simulink model "HPF_V01"  (R2018b)
settings: Solver=ode45  StartTime=0.0  StopTime=0.1  MaxStep=1e-6  RelTol=1e-3  EnableMultiTasking=on
libraries: fl_lib x18, nesl_utility x4, simulink x1
Description:
  | Inverting Op-Amp Circuit
  | 
  | This model shows a standard inverting op-amp circuit. The gain is given by -R2/R1, and
  | with the values set to R1=1K Ohm and R2=10K Ohm, the 0.1V peak-to-peak input
  | voltage is amplified to 1V peak-to-peak. As the Op-Amp block implements an ideal
  | (i.e. infinite gain) device, this gain is achieved regardless of output load.
  | 
  | 
  | Copyright 2008-2015 The MathWorks, Inc.
settings Model: ExtModeAutoUpdateStatusClock=off  Creator=MathWorks  LastModifiedBy=arkad
settings DataIOCC: LimitDataPoints=on  SaveFormat=Array  SignalLoggingSaveFormat=ModelDataLogs
settings OptimizationCC: ExpressionDepthLimit=2147483647  InitFltsAndDblsToZero=on  EfficientMapNaN2IntZero=off  LifeSpan=inf
settings DebuggingCC: SaveWithParameterizedLinksMsg=none  UnderspecifiedInitializationDetection=Classic  MergeDetectMultiDrivingBlocksExec=none  SignalResolutionControl=TryResolveAllWithWarning  SolverPrmCheckMsg=warning  FcnCallInpInsideContextMsg=warning  StateNameClashWarn=warning  SFUnexpectedBacktrackingDiag=warning  SFNoUnconditionalDefaultTransitionDiag=warning  SFExecutionAtInitializationDiag=none
settings HardwareCC: ProdBitPerPointer=32  ProdBitPerSizeT=32  ProdBitPerPtrDiffT=32  ProdLargestAtomicFloat=None  ProdIntDivRoundTo=Undefined  ProdEndianess=Unspecified  ProdWordSize=32  ProdHWDeviceType=32-bit Generic
settings ModelReferenceCC: PropagateSignalLabelsOutOfModel=off
settings SFSimCC: SimUseLocalCustomCode=off
settings RTWCC: RTWUseLocalCustomCode=off
settings CodeAppCC: StateflowObjectComments=on
settings GRTTargetCC: TargetFcnLib=ansi_tfl_tmw.mat  TargetLangStandard=C89/C90 (ANSI)  GeneratePreprocessorConditionals=Disable all  CombineOutputUpdateFcns=off  GRTInterface=on
settings ConfigComp: CovMetricSettings=dw  CovHtmlReporting=on  CovSaveCumulativeToWorkspaceVar=on  CovSaveSingleToWorkspaceVar=on  CovExternalEMLEnable=off
settings SimscapeCC: ExplicitSolverDiagnosticOptions=none  SimscapeNormalizeSystem=off

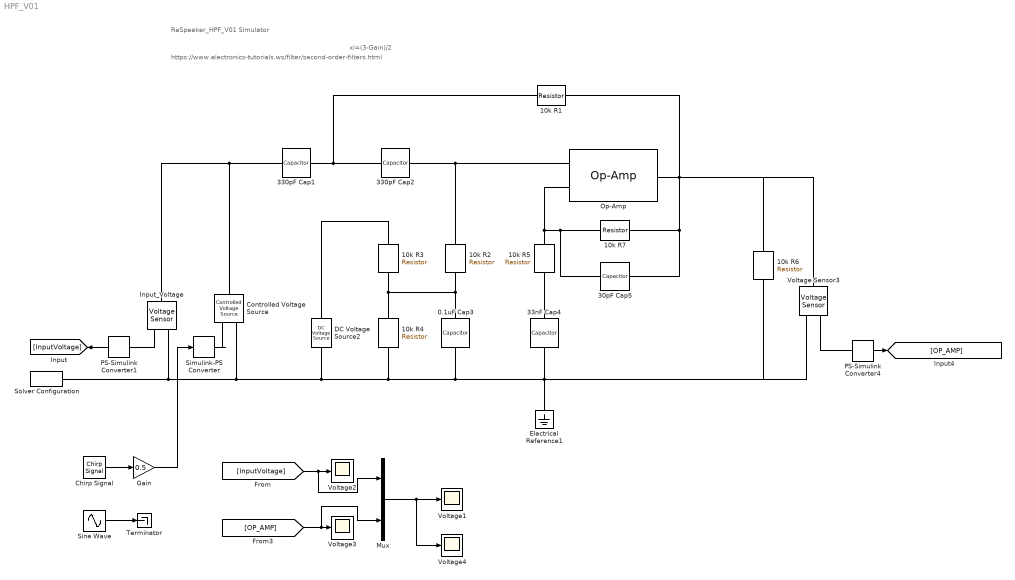
== system HPF_V01 ==
  note: https://www.electronics-tutorials.ws/filter/second-order-filters.html
  note: xi=(3-Gain)/2
  note: ReSpeaker_HPF_V01 Simulator
  0.1uF Cap3 : fl_lib/Electrical/Electrical Elements/Capacitor  c=0.1 uF  r=1e-6 Ohm  g=0 1/Ohm  i_specify=off  i_priority=None  i=0 A  i_nominal_specify=off  i_nominal_unit=A  i_nominal_value=1  v_specify=on  v_priority=None  v=2 V  v_nominal_specify=off  v_nominal_unit=V  v_nominal_value=1  vc_specify=off  vc_priority=High  vc=0 V  vc_nominal_specify=off  vc_nominal_unit=V  vc_nominal_value=1
  10k R{1..6} (6 alike) : fl_lib/Electrical/Electrical Elements/Resistor  R=10 kOhm  i_specify=off  i_priority=High  i=0 A  i_nominal_specify=off  i_nominal_unit=A  i_nominal_value=1  v_specify=off  v_priority=High  v=0 V  v_nominal_specify=off  v_nominal_unit=V  v_nominal_value=1
  10k R7 : fl_lib/Electrical/Electrical Elements/Resistor  R=18 kOhm  i_specify=off  i_priority=High  i=0 A  i_nominal_specify=off  i_nominal_unit=A  i_nominal_value=1  v_specify=off  v_priority=High  v=0 V  v_nominal_specify=off  v_nominal_unit=V  v_nominal_value=1
  30pF Cap5 : fl_lib/Electrical/Electrical Elements/Capacitor  c=30 pF  r=1e-6 Ohm  g=0 1/Ohm  i_specify=off  i_priority=None  i=0 A  i_nominal_specify=off  i_nominal_unit=A  i_nominal_value=1  v_specify=off  v_priority=None  v=0 V  v_nominal_specify=off  v_nominal_unit=V  v_nominal_value=1  vc_specify=off  vc_priority=High  vc=0 V  vc_nominal_specify=off  vc_nominal_unit=V  vc_nominal_value=1
  330pF Cap1 : fl_lib/Electrical/Electrical Elements/Capacitor  c=330 pF  r=1e-6 Ohm  g=0 1/Ohm  i_specify=off  i_priority=None  i=0 A  i_nominal_specify=off  i_nominal_unit=A  i_nominal_value=1  v_specify=off  v_priority=None  v=0 V  v_nominal_specify=off  v_nominal_unit=V  v_nominal_value=1  vc_specify=off  vc_priority=High  vc=0 V  vc_nominal_specify=off  vc_nominal_unit=V  vc_nominal_value=1
  330pF Cap2 : fl_lib/Electrical/Electrical Elements/Capacitor  c=330 pF  r=1e-6 Ohm  g=0 1/Ohm  i_specify=off  i_priority=None  i=0 A  i_nominal_specify=off  i_nominal_unit=A  i_nominal_value=1  v_specify=off  v_priority=None  v=0 V  v_nominal_specify=off  v_nominal_unit=V  v_nominal_value=1  vc_specify=off  vc_priority=High  vc=0 V  vc_nominal_specify=off  vc_nominal_unit=V  vc_nominal_value=1
  33nF Cap4 : fl_lib/Electrical/Electrical Elements/Capacitor  c=33 nF  r=1e-6 Ohm  g=0 1/Ohm  i_specify=off  i_priority=None  i=0 A  i_nominal_specify=off  i_nominal_unit=A  i_nominal_value=1  v_specify=off  v_priority=None  v=0 V  v_nominal_specify=off  v_nominal_unit=V  v_nominal_value=1  vc_specify=off  vc_priority=High  vc=0 V  vc_nominal_specify=off  vc_nominal_unit=V  vc_nominal_value=1
  Chirp Signal : simulink/Sources/Chirp Signal  f1=1000  T=0.1  f2=100000
  Controlled Voltage Source : fl_lib/Electrical/Electrical Sources/Controlled Voltage Source
  DC Voltage Source2 : fl_lib/Electrical/Electrical Sources/DC Voltage Source  v0=4 V
  Electrical Reference1 : fl_lib/Electrical/Electrical Elements/Electrical Reference
  Gain : Gain  Gain=0.5
  Input_Voltage : fl_lib/Electrical/Electrical Sensors/Voltage Sensor
  Mux : Mux  Inputs=2
  "Op-Amp " : fl_lib/Electrical/Electrical Elements/Op-Amp  outI_specify=off  outI_priority=High  outI=0 A  outI_nominal_specify=off  outI_nominal_unit=A  outI_nominal_value=1
  PS-Simulink Converter1 : nesl_utility/PS-Simulink Converter  PhysicalDomain=network_engine_domain  SubClassName=ps_output  LeftPortType=input  RightPortType=output  PseudoPeriodic=off  Frequencies=[]  Unit=1  AffineConversion=off
  PS-Simulink Converter4 : nesl_utility/PS-Simulink Converter  PhysicalDomain=network_engine_domain  SubClassName=ps_output  LeftPortType=input  RightPortType=output  PseudoPeriodic=off  Frequencies=[]  Unit=1  AffineConversion=off
  Simulink-PS Converter : nesl_utility/Simulink-PS Converter  PhysicalDomain=network_engine_domain  SubClassName=ps_input  LeftPortType=input  RightPortType=output  PseudoPeriodic=off  Frequencies=[]  NoiseDistribution=none  NoiseParameters=[]  Unit=1  AffineConversion=off  FilteringAndDerivatives=provide  SimscapeFilterOrder=1  InputFilterTimeConstant=0.001  UdotUserProvided=0
  Sine Wave : Sin  Amplitude=0.5  Frequency=50000*57.2958
  Solver Configuration : nesl_utility/Solver Configuration  PhysicalDomain=network_engine_domain  SubClassName=solver  LeftPortType=input  RightPortType=generic  Tones=[]  Harmonics=[]  SimulateNoise=off  Profile=off  UseLocalSampling=off  EnableSwitchedLinearOptims=on  FrequencyDomain=off  UseCCode=off  RelTol=0.001  AbsTol=1e-06  MinStep=1e-09  ToWorkspace=off  RevertToSquareIcSolve=off  NumHomotopyIterations=100  PhasorMode=off  PhasorModeNumHarmonics=1  DoDC=on  ResidualTolerance=1e-9  UseLocalSolver=on  LocalSolverChoice=NE_BACKWARD_EULER_ADVANCER  LocalSolverSampleTime=.00000001  DoFixedCost=on  MaxNonlinIter=3  MaxModeIter=2  LinearAlgebra=Sparse  EquationFormulation=NE_TIME_EF  DelaysMemoryBudget=1024  AutomaticFiltering=on  FilteringTimeConstant=0.000001  PartitionStorageMethod=AS_NEEDED  PartitionMemoryBudget=1024
  Terminator : Terminator
  Voltage Sensor3 : fl_lib/Electrical/Electrical Sensors/Voltage Sensor
  Voltage{1..4} (4 alike) : Scope
  wires:
  Mux/1 -> Voltage4/1, Voltage1/1
  PS-Simulink Converter1/1 -> [InputVoltage]
  [InputVoltage] -> Mux/1, Voltage2/1
  [OP_AMP] -> Mux/2, Voltage3/1
  PS-Simulink Converter4/1 -> [OP_AMP]
  Chirp Signal/1 -> Gain/1
  Gain/1 -> Simulink-PS Converter/1
  Sine Wave/1 -> Terminator/1
  connections:
  Solver Configuration/RConn1 -- Input_Voltage/RConn2 -- Controlled Voltage Source/RConn2 -- DC Voltage Source2/RConn1 -- 10k R4/RConn1 -- 0.1uF Cap3/RConn1 -- 10k R6/RConn1 -- Voltage Sensor3/RConn2 -- 33nF Cap4/RConn1 -- Electrical Reference1/LConn1
  Input_Voltage/RConn1 -- PS-Simulink Converter1/LConn1
  Controlled Voltage Source/LConn1 -- 330pF Cap1/LConn1 -- Input_Voltage/LConn1
  PS-Simulink Converter4/LConn1 -- Voltage Sensor3/RConn1
  Simulink-PS Converter/RConn1 -- Controlled Voltage Source/RConn1
  "Op-Amp "/LConn1 -- 10k R2/LConn1 -- 330pF Cap2/RConn1
  330pF Cap1/RConn1 -- 10k R1/LConn1 -- 330pF Cap2/LConn1
  DC Voltage Source2/LConn1 -- 10k R3/LConn1
  "Op-Amp "/RConn1 -- 10k R1/RConn1 -- Voltage Sensor3/LConn1 -- 10k R6/LConn1 -- 10k R7/RConn1 -- 30pF Cap5/RConn1
  10k R7/LConn1 -- 30pF Cap5/LConn1 -- 10k R5/LConn1 -- "Op-Amp "/LConn2
  10k R3/RConn1 -- 0.1uF Cap3/LConn1 -- 10k R2/RConn1 -- 10k R4/LConn1
  10k R5/RConn1 -- 33nF Cap4/LConn1
